simulink model "test_observer"  (R2019b)
settings: Solver=VariableStepAuto  StartTime=0.0  StopTime=15  MaxStep=1e-3  RelTol=1e-3
values from neighbouring files (symbols this model uses):
  A = [0 1;[-k -h]/m]    [esempio.m]
  Ac = [Ao-Bo*[K 0]-L*Co Bo*H;-Co 0]    [esempio.m]
  Ao = [A -B;zeros(1,n) 0]    [esempio.m]
  B = [0;1/m]    [esempio.m]
  Bc = [[0;0;0;1] [L;0]]    [esempio.m]
  Bo = [B;0]    [esempio.m]
  C = [1 0]    [esempio.m]
  Cc = [-[K 0] H]    [esempio.m]
  Ce = tmp(2)    [esempio.m]
  Co = [C 0]    [esempio.m]
  Cr = tmp(1)    [esempio.m]
  D = 0    [esempio.m]
  Dc = [0 0]    [esempio.m]
  H = -Ka(n+1:end)    [esempio.m]
  K = Ka(1:n)    [esempio.m]
undefined symbols (not defined in the file or in its folder): L
libraries: cstblocks x2
settings Model: Creator=jacobi  LastModifiedBy=jacobi

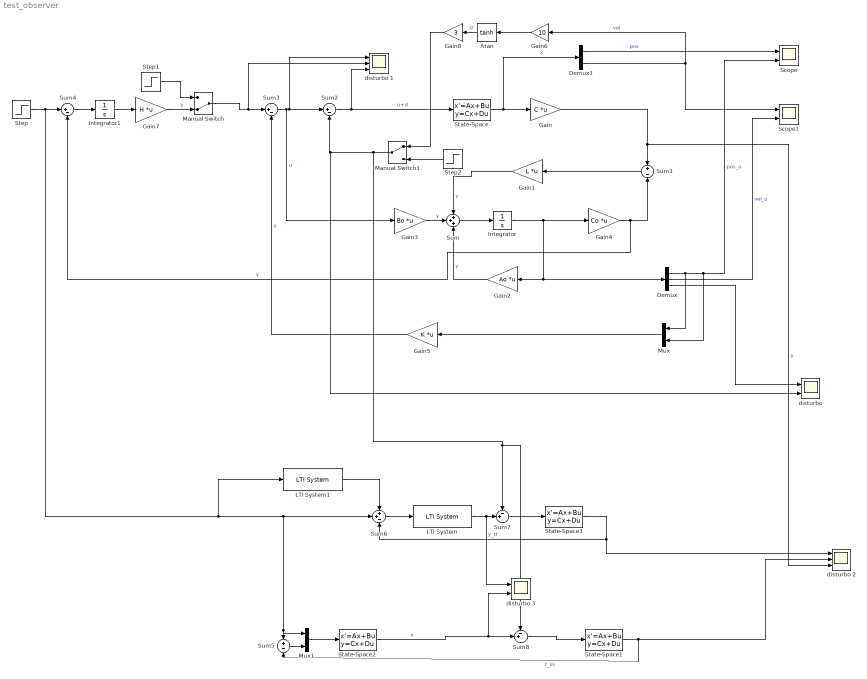
== system test_observer ==
  Atan : Trigonometry  Operator=tanh
  Demux : Demux  Outputs=3
  Demux1 : Demux  Outputs=2
  Gain : Gain  Gain=C  Multiplication=Matrix(K*u)
  Gain1 : Gain  Gain=L  Multiplication=Matrix(K*u)
  Gain2 : Gain  Gain=Ao  Multiplication=Matrix(K*u)
  Gain3 : Gain  Gain=Bo  Multiplication=Matrix(K*u)
  Gain4 : Gain  Gain=Co  Multiplication=Matrix(K*u)
  Gain5 : Gain  Gain=K  Multiplication=Matrix(K*u)
  Gain6 : Gain  Gain=10
  Gain7 : Gain  Gain=H  Multiplication=Matrix(K*u)
  Gain8 : Gain  Gain=3
  Integrator : Integrator
  Integrator1 : Integrator
  LTI System : cstblocks/LTI System  sys=Ce  IC=[]
  LTI System1 : cstblocks/LTI System  sys=Cr/Ce  IC=[]
  Manual Switch : ManualSwitch  CurrentSetting=0
  Manual Switch1 : ManualSwitch
  Mux : Mux  Inputs=2
  Mux1 : Mux  Inputs=2
  Scope : Scope  NumInputPorts=2
  Scope1 : Scope  NumInputPorts=2
  State-Space : StateSpace  A=A  B=B*1.5  C=eye(2)  D=[0;0]  InitialCondition=0
  State-Space1 : StateSpace  A=A  B=B  C=C  D=D  InitialCondition=0
  State-Space2 : StateSpace  A=Ac  B=Bc*[1 0;1 -1]  C=Cc  D=Dc*[1 0;1 -1]  InitialCondition=0
  State-Space3 : StateSpace  A=A  B=B  C=C  D=D  InitialCondition=0
  Step : Step  Time=5  After=0.1  SampleTime=0
  Step1 : Step  Time=5  SampleTime=0
  Step2 : Step  SampleTime=0
  Sum : Sum  Inputs=+++
  Sum1 : Sum  Inputs=+-
  Sum2 : Sum  Inputs=|+-
  Sum3 : Sum  Inputs=|+-
  Sum4 : Sum  Inputs=|+-
  Sum5 : Sum  Inputs=+-
  Sum6 : Sum  Inputs=++-
  Sum7 : Sum  Inputs=-+|
  Sum8 : Sum  Inputs=-+|
  "disturbo " : Scope  NumInputPorts=2
  disturbo 1 : Scope  NumInputPorts=3
  disturbo 2 : Scope  NumInputPorts=3
  disturbo 3 : Scope  NumInputPorts=2
  wires:
  State-Space/1 -> Demux1/1, Gain/1  "x"
  Gain/1 -> disturbo 2/3, Sum1/1  "y"
  Gain1/1 -> Sum/1  "y"
  Gain3/1 -> Sum/2  "y"
  Gain2/1 -> Sum/3  "y"
  Sum/1 -> Integrator/1
  Integrator/1 -> Gain2/1, Demux/1, Gain4/1
  Gain4/1 -> Sum1/2, Sum4/2  "y"
  Sum1/1 -> Gain1/1
  Demux1/1 -> Scope/1  "pos"
  Demux/1 -> Mux/1, Mux/2, Scope/2  "pos_o"
  Demux1/2 -> Gain6/1, Scope1/1  "vel"
  Demux/2 -> Scope1/2  "vel_o"
  Demux/3 -> "disturbo "/1
  Sum2/1 -> disturbo 1/3, State-Space/1  "u+d"
  Gain5/1 -> Sum3/2  "y"
  Sum3/1 -> Gain3/1, disturbo 1/1, Sum2/1  "u"
  Mux/1 -> Gain5/1
  Gain6/1 -> Atan/1
  Gain7/1 -> Manual Switch/2  "y"
  Integrator1/1 -> Gain7/1
  Sum4/1 -> Integrator1/1
  Step/1 -> LTI System1/1, Mux1/1, Sum5/1, Sum6/2, Sum4/1
  Manual Switch/1 -> disturbo 1/2, Sum3/1
  Step1/1 -> Manual Switch/1
  Atan/1 -> Gain8/1  "d"
  Step2/1 -> Manual Switch1/2
  State-Space1/1 -> disturbo 2/2, Sum5/2  "t_ss"
  Mux1/1 -> State-Space2/1
  Sum5/1 -> Mux1/2
  LTI System/1 -> disturbo 3/1, Sum7/2
  LTI System1/1 -> Sum6/1
  Sum6/1 -> LTI System/1
  State-Space3/1 -> disturbo 2/1, Sum6/3  "y_tf"
  Sum7/1 -> State-Space3/1
  Manual Switch1/1 -> "disturbo "/2, Sum2/2, Sum8/1, Sum7/1
  Sum8/1 -> State-Space1/1
  State-Space2/1 -> disturbo 3/2, Sum8/2  "x"
  Gain8/1 -> Manual Switch1/1
